simulink model "CRC4BitCheckSum"  (Simulink 8.3)
settings: Solver=ode45  StartTime=0.0  StopTime=10.0  RelTol=1e-3
libraries: simulink x6
settings Model: Creator=ohc  LastModifiedBy=ohc
settings DataIOCC: SignalLoggingSaveFormat=Dataset
settings DebuggingCC: UnderspecifiedInitializationDetection=Simplified  StateNameClashWarn=none
settings GRTTargetCC: CombineOutputUpdateFcns=on  GRTInterface=off

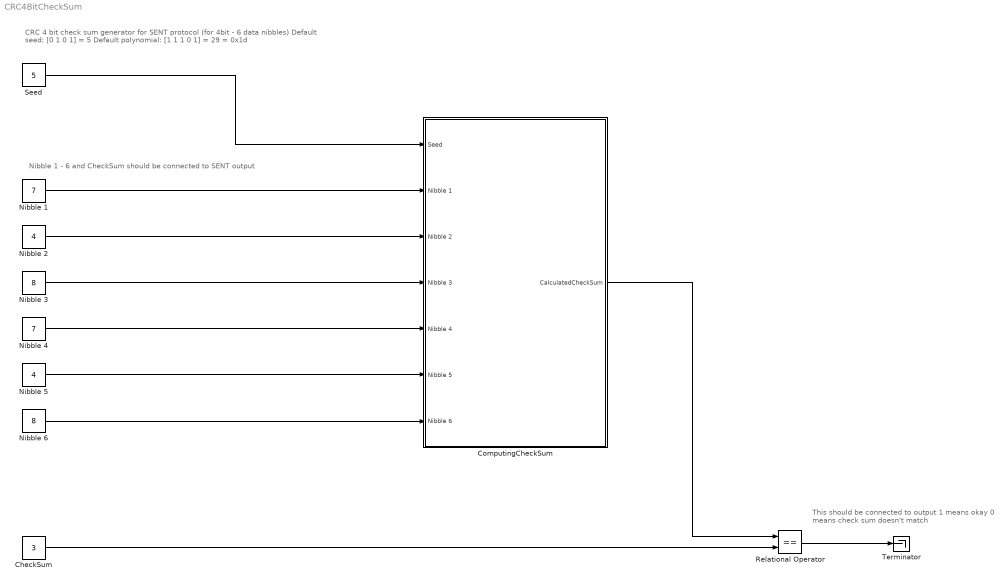
== system CRC4BitCheckSum ==
  note: CRC 4 bit check sum generator for SENT protocol (for 4bit - 6 data nibbles)
      | Default seed:  [0 1 0 1] = 5
      | Default polynomial: [1 1 1 0 1] =  29 = 0x1d
  note: This should be connected to output
      | 1 means okay 0 means check sum doesn't match
  note: Nibble 1 - 6 and CheckSum should be connected to SENT output
  CheckSum : Constant  Value=3  OutDataTypeStr=uint8
  ComputingCheckSum : Subsystem
  Nibble 1 : Constant  Value=7  OutDataTypeStr=uint8
  Nibble 2 : Constant  Value=4  OutDataTypeStr=uint8
  Nibble 3 : Constant  Value=8  OutDataTypeStr=uint8
  Nibble 4 : Constant  Value=7  OutDataTypeStr=uint8
  Nibble 5 : Constant  Value=4  OutDataTypeStr=uint8
  Nibble 6 : Constant  Value=8  OutDataTypeStr=uint8
  Relational Operator : RelationalOperator  Operator===  OutDataTypeStr=boolean
  Seed : Constant  Value=5  OutMin=0  OutMax=15  OutDataTypeStr=uint8
  Terminator : Terminator
  wires:
  Seed/1 -> ComputingCheckSum/1(Seed)
  Nibble 1/1 -> ComputingCheckSum/2(Nibble 1)
  Nibble 2/1 -> ComputingCheckSum/3(Nibble 2)
  Nibble 3/1 -> ComputingCheckSum/4(Nibble 3)
  Nibble 4/1 -> ComputingCheckSum/5(Nibble 4)
  Nibble 5/1 -> ComputingCheckSum/6(Nibble 5)
  Nibble 6/1 -> ComputingCheckSum/7(Nibble 6)
  CheckSum/1 -> Relational Operator/2
  ComputingCheckSum/1(CalculatedCheckSum) -> Relational Operator/1
  Relational Operator/1 -> Terminator/1

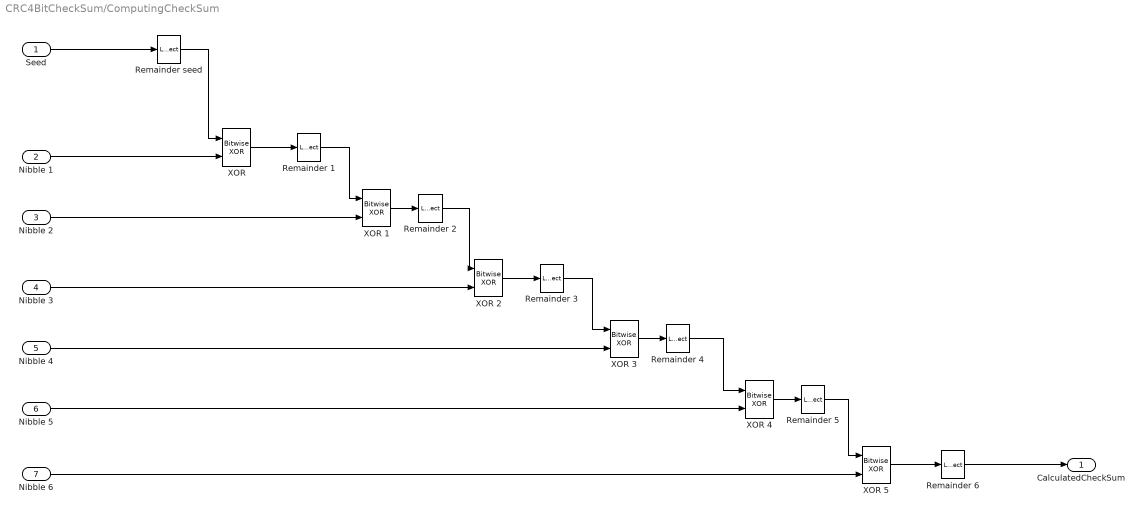
== system CRC4BitCheckSum/ComputingCheckSum ==
  Seed : Inport
  Nibble 1 : Inport  Port=2
  Nibble 2 : Inport  Port=3
  Nibble 3 : Inport  Port=4
  Nibble 4 : Inport  Port=5
  Nibble 5 : Inport  Port=6
  Nibble 6 : Inport  Port=7
  Remainder {1,3..6} (5 alike) : LookupNDDirect  NumberOfTableDimensions=1  Table=[0 13 7 10 14 3 9 4 1 12 6 11 15 2 8 5 ]  TableMin=0  TableMax=15  TableDataTypeStr=uint8
  Remainder 2 : LookupNDDirect  NumberOfTableDimensions=1  Table=[0,13,7,10,14,3,9,4,1,12,6,11,15,2,8,5]  TableMin=0  TableMax=15  TableDataTypeStr=uint8
  Remainder seed : LookupNDDirect  NumberOfTableDimensions=1  Table=[0 13 7 10 14 3 9 4 1 12 6 11 15 2 8 5 ]  TableMin=0  TableMax=15  TableDataTypeStr=uint8
  XOR {,1..5} (6 alike) : simulink/Logic and Bit Operations/Bitwise Operator  logicop=XOR  UseBitMask=off  NumInputPorts=2  BitMask=bin2dec('11011001')  BitMaskRealWorld=Stored Integer
  CalculatedCheckSum : Outport
  wires:
  Nibble 3/1 -> XOR 2/2
  Remainder 6/1 -> CalculatedCheckSum/1
  Remainder 4/1 -> XOR 4/1
  XOR 5/1 -> Remainder 6/1
  Remainder 5/1 -> XOR 5/1
  Nibble 6/1 -> XOR 5/2
  XOR 1/1 -> Remainder 2/1
  Nibble 1/1 -> "XOR "/2
  Seed/1 -> Remainder seed/1
  Remainder seed/1 -> "XOR "/1
  Remainder 2/1 -> XOR 2/1
  Nibble 4/1 -> XOR 3/2
  Nibble 5/1 -> XOR 4/2
  XOR 2/1 -> Remainder 3/1
  Remainder 1/1 -> XOR 1/1
  XOR 3/1 -> Remainder 4/1
  XOR 4/1 -> Remainder 5/1
  Nibble 2/1 -> XOR 1/2
  Remainder 3/1 -> XOR 3/1
  "XOR "/1 -> Remainder 1/1
